simulink model "Simulink"  (R2022b)
settings: Solver=ode4  StartTime=0.0  StopTime=20  FixedStep=0.001  RelTol=1e-3
PreLoadFcn:
  | Bsm = 0.01;
  | Bsf = 1.5;
  | Jm = 0.002;
  | Jgear1= 0.001;
  | Jf= 0.0204;
  | Gc = 9.95;
  | GR = 1.7;
  | Ke = 0.35;
  | Kf = 0.5;
  | Kg = 2.0;
  | Kr= 0.9;
  | Ks= 0.9;
  | Kt = 0.35;
  | L = 0.1;
  | Lf = 0.35;
  | Mf = 0.5;
  | R = 4;
  | g = 9.81;
  | theta_U = deg2rad(5);
  | theta_Fref = deg2rad(55);
settings Model: Creator=Jalal  LastModifiedBy=Jalal
settings DataIOCC: SaveFormat=Array  ReturnWorkspaceOutputs=off

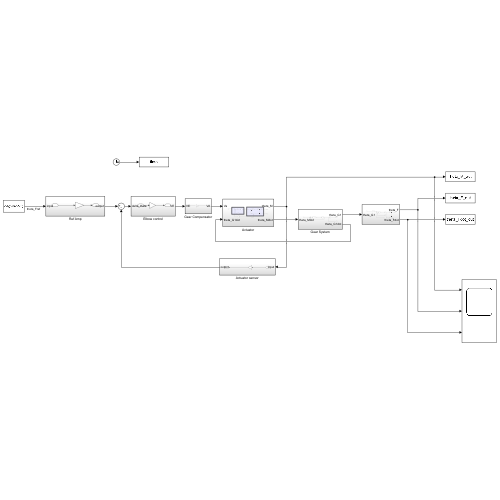
[thumbnail: Simulink's stored preview of the top-level diagram]
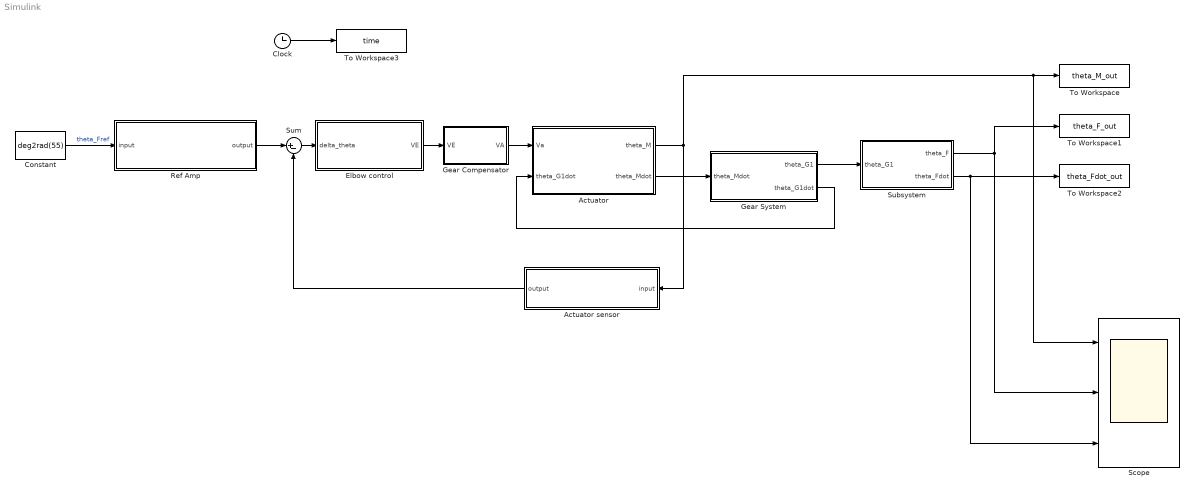
== system Simulink ==
  Actuator : Subsystem
  Actuator sensor : Subsystem
  Clock : Clock
  Constant : Constant  Value=deg2rad(55)  VectorParams1D=off
  Elbow control : Subsystem
  Gear Compensator : Subsystem
  Gear System : Subsystem
  Ref Amp : Subsystem
  Scope : Scope  NumInputPorts=3
  Subsystem : Subsystem
  Sum : Sum  Inputs=|+-
  To Workspace : ToWorkspace  VariableName=theta_M_out  SampleTime=-1
  To Workspace1 : ToWorkspace  VariableName=theta_F_out  SampleTime=-1
  To Workspace2 : ToWorkspace  VariableName=theta_Fdot_out  SampleTime=-1
  To Workspace3 : ToWorkspace  VariableName=time  SampleTime=-1
  wires:
  Gear System/1(theta_G1) -> Subsystem/1(theta_G1)
  Subsystem/1(theta_F) -> To Workspace1/1, Scope/2
  Subsystem/2(theta_Fdot) -> To Workspace2/1, Scope/3
  Actuator/1(theta_M) -> Scope/1, To Workspace/1, Actuator sensor/1(input)
  Gear System/2(theta_G1dot) -> Actuator/2(theta_G1dot)
  Actuator/2(theta_Mdot) -> Gear System/1(theta_Mdot)
  Actuator sensor/1(output) -> Sum/2
  Constant/1 -> Ref Amp/1(input)  "theta_Fref"
  Ref Amp/1(output) -> Sum/1
  Gear Compensator/1(VA) -> Actuator/1(Va)
  Elbow control/1(VE) -> Gear Compensator/1(VE)
  Sum/1 -> Elbow control/1(delta_theta)
  Clock/1 -> To Workspace3/1

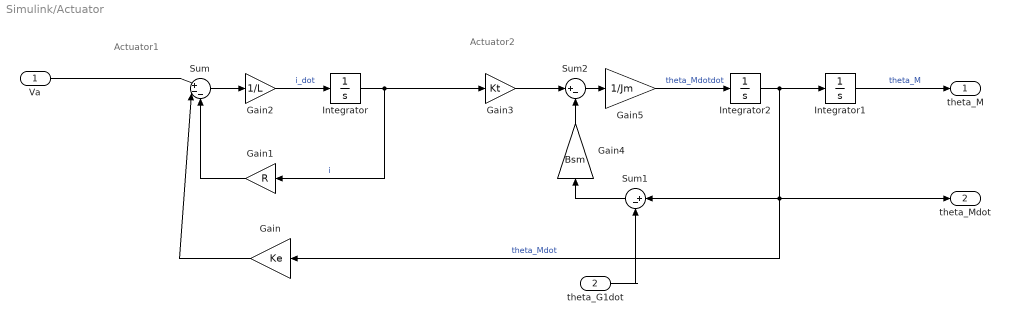
== system Simulink/Actuator ==
  note: Actuator2
  note: Actuator1
  Va : Inport
  theta_G1dot : Inport  Port=2
  Gain : Gain  Gain=Ke
  Gain1 : Gain  Gain=R
  Gain2 : Gain  Gain=1/L
  Gain3 : Gain  Gain=Kt
  Gain4 : Gain  Gain=Bsm
  Gain5 : Gain  Gain=1/Jm
  Integrator : Integrator
  Integrator1 : Integrator
  Integrator2 : Integrator
  Sum : Sum  Inputs=|+--
  Sum1 : Sum  Inputs=|+-
  Sum2 : Sum  Inputs=|+-
  theta_M : Outport
  theta_Mdot : Outport  Port=2
  wires:
  Gain/1 -> Sum/2
  Gain2/1 -> Integrator/1  "i_dot"
  Integrator/1 -> Gain3/1, Gain1/1  "i"
  Sum/1 -> Gain2/1
  Va/1 -> Sum/1
  Gain1/1 -> Sum/3
  Gain4/1 -> Sum2/2
  Gain3/1 -> Sum2/1
  Sum2/1 -> Gain5/1
  Integrator1/1 -> theta_M/1  "theta_M"
  Sum1/1 -> Gain4/1
  theta_G1dot/1 -> Sum1/2
  Integrator2/1 -> theta_Mdot/1, Gain/1, Sum1/1, Integrator1/1  "theta_Mdot"
  Gain5/1 -> Integrator2/1  "theta_Mdotdot"

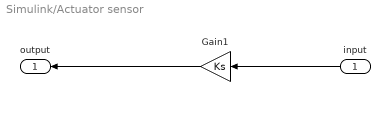
== system Simulink/Actuator sensor ==
  input : Inport
  Gain1 : Gain  Gain=Ks
  output : Outport
  wires:
  input/1 -> Gain1/1
  Gain1/1 -> output/1

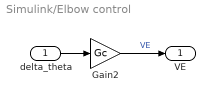
== system Simulink/Elbow control ==
  delta_theta : Inport
  Gain2 : Gain  Gain=Gc
  VE : Outport
  wires:
  Gain2/1 -> VE/1  "VE"
  delta_theta/1 -> Gain2/1

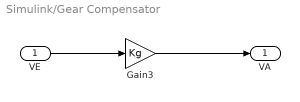
== system Simulink/Gear Compensator ==
  VE : Inport
  Gain3 : Gain  Gain=Kg
  VA : Outport
  wires:
  VE/1 -> Gain3/1
  Gain3/1 -> VA/1

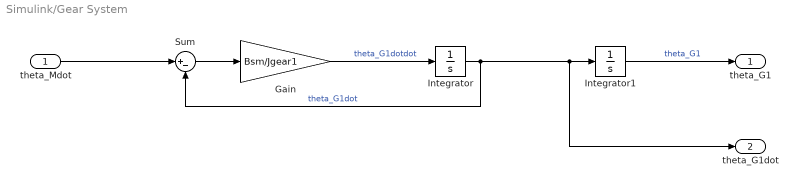
== system Simulink/Gear System ==
  theta_Mdot : Inport
  Gain : Gain  Gain=Bsm/Jgear1
  Integrator : Integrator
  Integrator1 : Integrator
  Sum : Sum  Inputs=|+-
  theta_G1 : Outport
  theta_G1dot : Outport  Port=2
  wires:
  Integrator1/1 -> theta_G1/1  "theta_G1"
  Sum/1 -> Gain/1
  theta_Mdot/1 -> Sum/1
  Gain/1 -> Integrator/1  "theta_G1dotdot"
  Integrator/1 -> Sum/2, theta_G1dot/1, Integrator1/1  "theta_G1dot"

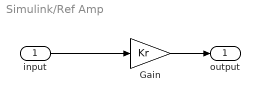
== system Simulink/Ref Amp ==
  input : Inport
  Gain : Gain  Gain=Kr
  output : Outport
  wires:
  input/1 -> Gain/1
  Gain/1 -> output/1

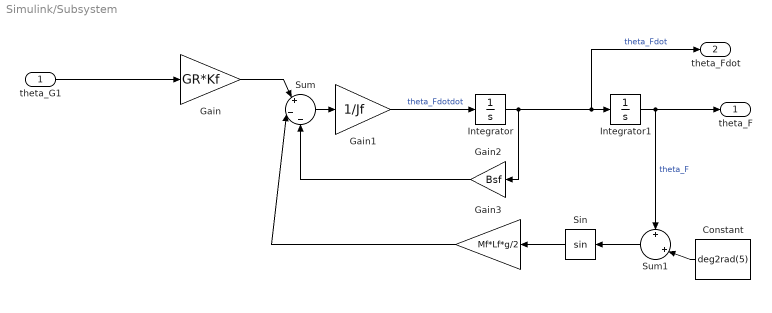
== system Simulink/Subsystem ==
  theta_G1 : Inport
  Constant : Constant  Value=deg2rad(5)
  Gain : Gain  Gain=GR*Kf
  Gain1 : Gain  Gain=1/Jf
  Gain2 : Gain  Gain=Bsf
  Gain3 : Gain  Gain=Mf*Lf*g/2
  Integrator : Integrator
  Integrator1 : Integrator  InitialCondition=deg2rad(-9)
  Sin : Trigonometry  OutputSignalType=real
  Sum : Sum  Inputs=|+|-|-
  Sum1 : Sum  Inputs=+|+|
  theta_F : Outport
  theta_Fdot : Outport  Port=2
  wires:
  Sin/1 -> Gain3/1
  Gain2/1 -> Sum/3
  Gain3/1 -> Sum/2
  Integrator1/1 -> theta_F/1, Sum1/1  "theta_F"
  Gain/1 -> Sum/1
  Integrator/1 -> Gain2/1, theta_Fdot/1, Integrator1/1  "theta_Fdot"
  Sum/1 -> Gain1/1
  Gain1/1 -> Integrator/1  "theta_Fdotdot"
  Constant/1 -> Sum1/2
  Sum1/1 -> Sin/1
  theta_G1/1 -> Gain/1
